simulink model "model"  (R2023a)
settings: Solver=VariableStepAuto  StartTime=0.0  StopTime=10.0  MaxStep=.0001  RelTol=1e-3
values from neighbouring files (symbols this model uses):
  B = 0.0001    [parameters.m]
  F = 50    [parameters.m]
  J = 0.00015    [parameters.m]
  Lambda_m = 0.193    [parameters.m]
  Lds = .114    (= 0.114)    [parameters.m]
  Lqs = .075    (= 0.075)    [parameters.m]
  P = 4    [parameters.m]
  Rs = 2.48    [parameters.m]
  Vph_p = 220*sqrt(2)    [parameters.m]
libraries: spsControlledVoltageSourceLib x3, spsPermanentMagnetSynchronousMachineLib x1, spsabctoAlphaBetaZeroLib x1, sps_lib x1
settings Model: Creator=User  LastModifiedBy=User

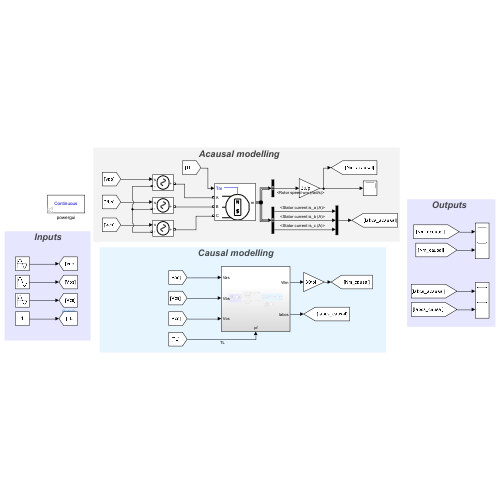
[thumbnail: Simulink's stored preview of the top-level diagram]
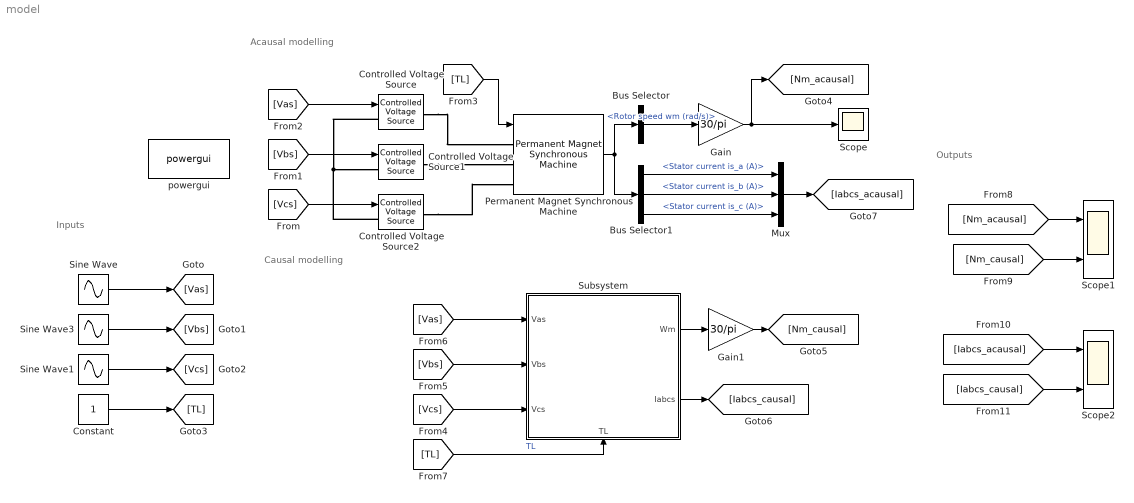
== system model ==
  note: Causal modelling
  note: Acausal modelling
  note: Inputs
  note: Outputs
  Bus Selector : BusSelector  OutputSignals=Rotor speed wm (rad/s)
  Bus Selector1 : BusSelector  OutputSignals=Stator current is_a (A),Stator current is_b (A),Stator current is_c (A)
  Constant : Constant
  Controlled Voltage Source : spsControlledVoltageSourceLib/Controlled Voltage Source  Initialize=on  Source_Type=AC  Amplitude=0  Phase=0  Frequency=0  Measurements=None
  Controlled Voltage Source1 : spsControlledVoltageSourceLib/Controlled Voltage Source  Initialize=on  Source_Type=AC  Amplitude=0  Phase=0  Frequency=0  Measurements=None
  Controlled Voltage Source2 : spsControlledVoltageSourceLib/Controlled Voltage Source  Initialize=on  Source_Type=AC  Amplitude=0  Phase=0  Frequency=0  Measurements=None
  Gain : Gain  Gain=30/pi
  Gain1 : Gain  Gain=30/pi
  Mux : Mux  Inputs=3
  Permanent Magnet Synchronous Machine : spsPermanentMagnetSynchronousMachineLib/Permanent Magnet Synchronous Machine  NbPhases=3  FluxDistribution=Sinusoidal  RotorType=Salient-pole  MechanicalLoad=Torque Tm  PresetModel=No  ShowDetailedParameters=on  MeasurementBus=off  Resistance=Rs  Inductance=8.5e-3  dqInductances=[Lds,Lqs]  La=La  MachineConstant=Flux linkage established by magnets (V.s)  Flux=Lambda_m  VoltageCst=70.0127  TorqueCst=0.579  Flat=120  Mechanical=[J B P/2 0]  PolePairs=4  InitialConditions=[0,0, 0,0]  InitialConditions5ph=[0 0 0 0 0 0]  RefAngle=Aligned with phase A axis (original Park)  IterativeDiscreteModel=Trapezoidal non iterative  TsBlock=-1  TsPowergui=0
  Scope : Scope
  Scope1 : Scope  NumInputPorts=2
  Scope2 : Scope  NumInputPorts=2
  Sine Wave : Sin  Amplitude=Vph_p  Frequency=2*pi*F  SampleTime=0
  Sine Wave1 : Sin  Amplitude=Vph_p  Frequency=2*pi*F  Phase=2*pi/3  SampleTime=0
  Sine Wave3 : Sin  Amplitude=Vph_p  Frequency=2*pi*F  Phase=-2*pi/3  SampleTime=0
  Subsystem : Subsystem
      settings: PortSchema="{\"entries\":[{\"content\":{\"sides\":[{\"content\":{\"connectorIds\":[\"In1\",\"In2\",\"In3\"]},\"type\":\"ConnectorPlacement.EquallySpacedRectSide\",\"uuid\":\"2d0cb5ef-c294-471d-8399-96b3c67f98e8\"},{\"content\":{\"connectorIds\":[\"Out1\",\"Out2\"],\"side\":\"RIGHT\"},\"type\":\"ConnectorPlacement.EquallySpacedRectSide\",\"uuid\":\"760ac53b-deac-4a80-bd19-ac013c03b708\"},{\"content\":{\"side\":\"TOP\"},\"type\":\"ConnectorPlacement.EquallySpacedRectSide\",\"uuid\":\"992570c0-27bb-47e0-9b33-abce524ec118\"},{\"content\":{\"connectorIds\":[\"In4\"],\"side\":\"BOTTOM\"},\"type\":\"ConnectorPlacement.EquallySpacedRectSide\",\"uuid\":\"4948debc-1d59-459c-9ab0-941c046a6db6\"}]},\"type\":\"ConnectorPlacement.EquallySpacedConnector\",\"uuid\":\"3b9b5ce2-f2fc-4c41-8b06-1a8949cdc782\"}],\"packageUris\":[\"http://schema.mathworks.com/mf0/Connector/R2020b\"],\"version\":\"1.0\"}"
  powergui : sps_lib/powergui  Priority=1  SimulationMode=Continuous  SampleTime=50e-6  frequency=60  Iterations=50  frequencyindice=0  Pbase=100e6  ErrMax=1e-4  UnitsV=kV  UnitsW=MW  buscounter=0  FunctionMessages=off  echomessages=off  EnableUseOfTLC=off  CurrentSourceSwitches=off  DisableSnubberDevices=off  DisableRonSwitches=off  DisableVfSwitches=off  DisplayEquations=off  AutomaticDiscreteSolvers=off  SolverType=Tustin/Backward Euler (TBE)  Interpol=off  ExternalGateDelay=off  methode=off  Ts=100  x0status=blocks  SPID=on  SwTol=0  HookPort=off  NonlinearTolerance=1e-4  nMaxIteration=100  ContinueOnMaxIteration=off  RestoreLinks=warning  ResistiveCurrentMeasurement=off  Frange=[0:2:500]  Ylog=off  Xlog=on  ShowGrid=off  save=off  variable=ZData  structure=0  ZoomFFT=off  StartTime=0.0  cycles=1  DisplayStyle=1  fundamental=60  FreqAxis=off  MaxFrequency=1000  frequencyindicesteady=1  RmsSteady=1  display=off
  wires:
  Sine Wave/1 -> [Vas]
  Sine Wave3/1 -> [Vbs]
  Sine Wave1/1 -> [Vcs]
  Constant/1 -> [TL]
  [TL] -> Permanent Magnet Synchronous Machine/1
  [Vcs] -> Controlled Voltage Source2/1
  [Vbs] -> Controlled Voltage Source1/1
  [Vas] -> Controlled Voltage Source/1
  Permanent Magnet Synchronous Machine/1 -> Bus Selector/1, Bus Selector1/1
  Bus Selector/1 -> Gain/1  "<Rotor speed wm (rad/s)>"
  Gain/1 -> Scope/1, [Nm_acausal]
  [Vas] -> Subsystem/1(Vas)
  [Vbs] -> Subsystem/2(Vbs)
  [Vcs] -> Subsystem/3(Vcs)
  [TL] -> Subsystem/4(TL)  "TL"
  Subsystem/1(Wm) -> Gain1/1
  Gain1/1 -> [Nm_causal]
  [Nm_acausal] -> Scope1/1
  [Nm_causal] -> Scope1/2
  Subsystem/2(Iabcs) -> [Iabcs_causal]
  [Iabcs_acausal] -> Scope2/1
  [Iabcs_causal] -> Scope2/2
  Bus Selector1/1 -> Mux/1  "<Stator current is_a (A)>"
  Bus Selector1/2 -> Mux/2  "<Stator current is_b (A)>"
  Bus Selector1/3 -> Mux/3  "<Stator current is_c (A)>"
  Mux/1 -> [Iabcs_acausal]
  connections:
  Controlled Voltage Source/RConn1 -- Permanent Magnet Synchronous Machine/LConn1
  Controlled Voltage Source1/RConn1 -- Permanent Magnet Synchronous Machine/LConn2
  Controlled Voltage Source2/RConn1 -- Permanent Magnet Synchronous Machine/LConn3
  Controlled Voltage Source2/LConn1 -- Controlled Voltage Source/LConn1 -- Controlled Voltage Source1/LConn1

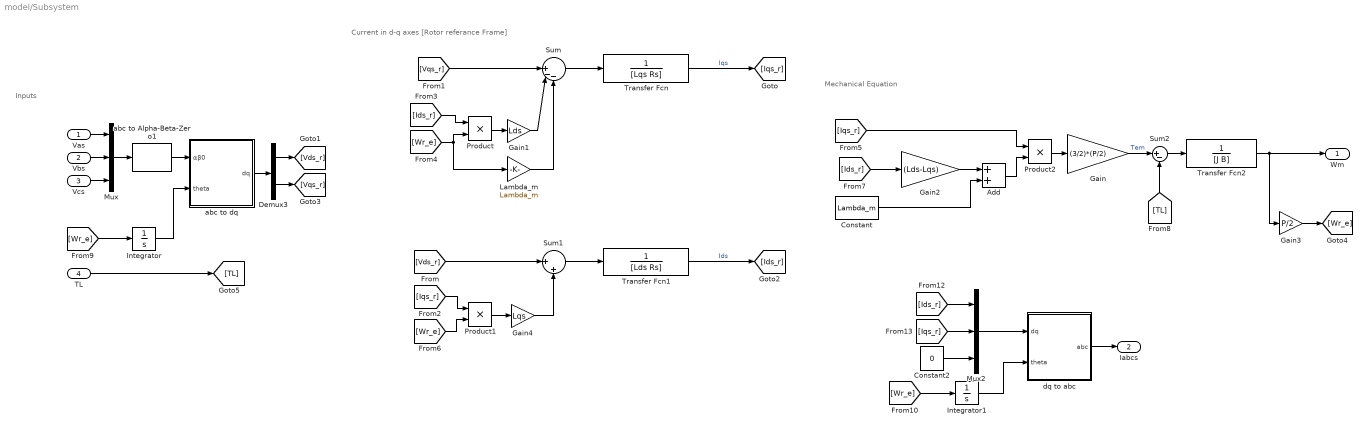
== system model/Subsystem ==
  note: Mechanical Equation
  note: Current in d-q axes [Rotor referance Frame]
  note: Inputs
  Vas : Inport
  Vbs : Inport  Port=2
  Vcs : Inport  Port=3
  TL : Inport  Port=4
  Add : Sum
  Constant : Constant  Value=Lambda_m
  Constant2 : Constant  Value=0
  Demux3 : Demux  Outputs=2
  Gain : Gain  Gain=(3/2)*(P/2)
  Gain1 : Gain  Gain=Lds
  Gain2 : Gain  Gain=(Lds-Lqs)
  Gain3 : Gain  Gain=P/2
  Gain4 : Gain  Gain=Lqs
  Integrator : Integrator
  Integrator1 : Integrator
  Lambda_m : Gain  Gain=Lambda_m
  Mux : Mux  Inputs=3
  Mux2 : Mux  Inputs=3
  Product : Product
  Product1 : Product
  Product2 : Product
  Sum : Sum  Inputs=||+--
  Sum1 : Sum  Inputs=||+|+
  Sum2 : Sum  Inputs=|+-
  Transfer Fcn : TransferFcn  Denominator=[Lqs Rs]
  Transfer Fcn1 : TransferFcn  Denominator=[Lds Rs]
  Transfer Fcn2 : TransferFcn  Denominator=[J B]
  abc to Alpha-Beta-Zero1 : spsabctoAlphaBetaZeroLib/abc to Alpha-Beta-Zero
  abc to dq : Subsystem
  dq to abc : Subsystem
  Wm : Outport
  Iabcs : Outport  Port=2
  wires:
  abc to Alpha-Beta-Zero1/1 -> abc to dq/1(αβ0)
  Demux3/1 -> [Vds_r]
  Mux/1 -> abc to Alpha-Beta-Zero1/1
  abc to dq/1(dq) -> Demux3/1
  Demux3/2 -> [Vqs_r]
  Vas/1 -> Mux/1
  Vbs/1 -> Mux/2
  Vcs/1 -> Mux/3
  [Vqs_r] -> Sum/1
  Sum/1 -> Transfer Fcn/1
  Transfer Fcn/1 -> [Iqs_r]  "Iqs"
  Transfer Fcn1/1 -> [Ids_r]  "Ids"
  Sum1/1 -> Transfer Fcn1/1
  [Vds_r] -> Sum1/1
  [Ids_r] -> Product/1
  [Wr_e] -> Product/2, Lambda_m/1
  Product/1 -> Gain1/1
  Gain1/1 -> Sum/2
  Lambda_m/1 -> Sum/3
  [Wr_e] -> Product1/2
  [Iqs_r] -> Product1/1
  Product1/1 -> Gain4/1
  [Ids_r] -> Gain2/1
  Gain2/1 -> Add/1
  Constant/1 -> Add/2
  Product2/1 -> Gain/1
  Add/1 -> Product2/2
  [Iqs_r] -> Product2/1
  Gain/1 -> Sum2/1  "Tem"
  TL/1 -> [TL]
  [TL] -> Sum2/2
  Sum2/1 -> Transfer Fcn2/1
  Transfer Fcn2/1 -> Wm/1, Gain3/1
  Gain3/1 -> [Wr_e]
  [Wr_e] -> Integrator/1
  Integrator/1 -> abc to dq/2(theta)
  Gain4/1 -> Sum1/2
  Mux2/1 -> dq to abc/1(dq)
  [Iqs_r] -> Mux2/2
  Integrator1/1 -> dq to abc/2(theta)
  dq to abc/1(abc) -> Iabcs/1
  Constant2/1 -> Mux2/3
  [Ids_r] -> Mux2/1
  [Wr_e] -> Integrator1/1

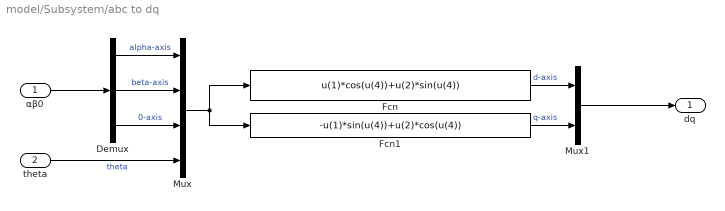
== system model/Subsystem/abc to dq ==
  αβ0 : Inport
  theta : Inport  Port=2
  Demux : Demux  Outputs=3
  Fcn : Fcn  Expr=u(1)*cos(u(4))+u(2)*sin(u(4))
  Fcn1 : Fcn  Expr=-u(1)*sin(u(4))+u(2)*cos(u(4))
  Mux : Mux
  Mux1 : Mux  Inputs=2
  dq : Outport
  wires:
  Mux/1 -> Fcn/1, Fcn1/1
  Fcn/1 -> Mux1/1  "d-axis"
  αβ0/1 -> Demux/1
  Demux/1 -> Mux/1  "alpha-axis"
  Demux/3 -> Mux/3  "0-axis"
  Demux/2 -> Mux/2  "beta-axis"
  theta/1 -> Mux/4  "theta"
  Fcn1/1 -> Mux1/2  "q-axis"
  Mux1/1 -> dq/1

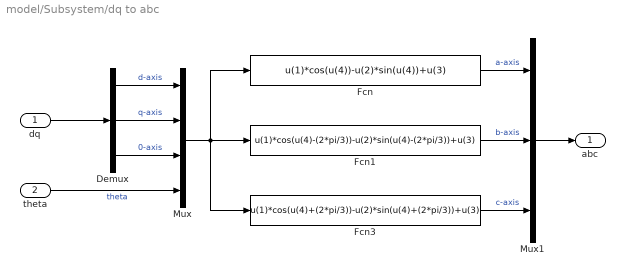
== system model/Subsystem/dq to abc ==
  dq : Inport
  theta : Inport  Port=2
  Demux : Demux  Outputs=3
  Fcn : Fcn  Expr=u(1)*cos(u(4))-u(2)*sin(u(4))+u(3)
  Fcn1 : Fcn  Expr=u(1)*cos(u(4)-(2*pi/3))-u(2)*sin(u(4)-(2*pi/3))+u(3)
  Fcn3 : Fcn  Expr=u(1)*cos(u(4)+(2*pi/3))-u(2)*sin(u(4)+(2*pi/3))+u(3)
  Mux : Mux
  Mux1 : Mux  Inputs=3
  abc : Outport
  wires:
  Fcn/1 -> Mux1/1  "a-axis"
  Fcn3/1 -> Mux1/3  "c-axis"
  dq/1 -> Demux/1
  Demux/1 -> Mux/1  "d-axis"
  Demux/3 -> Mux/3  "0-axis"
  Demux/2 -> Mux/2  "q-axis"
  theta/1 -> Mux/4  "theta"
  Mux/1 -> Fcn3/1, Fcn1/1, Fcn/1
  Fcn1/1 -> Mux1/2  "b-axis"
  Mux1/1 -> abc/1
